simulink model "ch6example12"  (Simulink 5.0)
settings: Solver=FixedStepDiscrete  StartTime=0.0  StopTime=10.0  FixedStep=1/8000  RelTol=1e-3
libraries: commutil2 x2, commsrccod2 x2, dspwin32 x2, dspbuff3 x1
settings Model: LastModifiedBy=shaoyubin

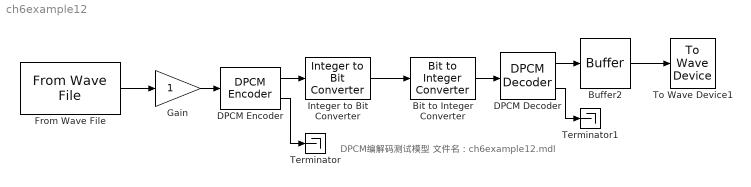
== system ch6example12 ==
  note: DPCM编解码测试模型
      | 文件名：ch6example12.mdl
  Bit to Integer Converter : commutil2/Bit to Integer Converter  nbits=4
  Buffer2 : dspbuff3/Buffer  N=512  V=0  ic=0
  DPCM Decoder : commsrccod2/DPCM Decoder  num="[0    0.9010   -0.0748   -0.0791   -0.0601    0.0598]"  den=1  codebook=[-15/16:2/16:15/16]  sample_time=1/8000
  DPCM Encoder : commsrccod2/DPCM Encoder  num="[0    0.9010   -0.0748   -0.0791   -0.0601    0.0598]"  den=1  partition=[-7/8:1/8:7/8]  codebook=[-15/16:2/16:15/16]  sample_time=1/8000
  From Wave File : dspwin32/From Wave File  FileName=./GDGvoice8000.wav  SamplesPerFrame=1  MinBufSize=512  dType=Double
  Gain : Gain  SaturateOnIntegerOverflow=on
  Integer to Bit Converter : commutil2/Integer to Bit Converter  nbits=4
  Terminator : Terminator
  Terminator1 : Terminator
  To Wave Device1 : dspwin32/To Wave Device  bufDuration=2  initDelay=0.1  useDefaultDevice=on  userDeviceID=SigmaTel C-Major Audio  enable24Bit=off
  wires:
  DPCM Encoder/1 -> Integer to Bit Converter/1
  From Wave File/1 -> Gain/1
  Gain/1 -> DPCM Encoder/1
  Buffer2/1 -> To Wave Device1/1
  DPCM Decoder/1 -> Buffer2/1
  DPCM Encoder/2 -> Terminator/1
  DPCM Decoder/2 -> Terminator1/1
  Integer to Bit Converter/1 -> Bit to Integer Converter/1
  Bit to Integer Converter/1 -> DPCM Decoder/1
